simulink model "slexIonosphereClassificationSVMPredictExample"  (R2021a)
settings: Solver=FixedStepDiscrete  StartTime=0.0  StopTime=radarReturnInput.time(end)  RelTol=1e-3
PreLoadFcn:
  | load ionosphere
  | 
  | prsntX = X(1:300,:);
  | prsntY = Y(1:300);
  | ftrX = X(301:end,:);
  | ftrY = Y(301:end);
  | 
  | svmMdl = fitcsvm(prsntX,prsntY,'Standardize',true);
  | 
  | radarReturnInput.time = (0:50)';
  | radarReturnInput.signals(1).values = ftrX;
  | radarReturnInput.signals(1).dimensions = size(ftrX,2);
values from neighbouring files (symbols this model uses):
  X = meas(:,1:2)    [ClusteringUsingGaussianMixtureModelsExample.m]    (also in ComputePairwiseDistance2UsingACustomDistanceFunctionExample.m = rand(3,3); EstimatePosteriorClassProbabilitiesECOCExample.m = X'; FittingGaussianProcessRegressionModelsToLargeDatasetsExample.m = [X,X.^2]; ModelswithCorrelatedandUncorrelatedRandomEffectsExample.m = [ones(406,1) Acceleration Horsepower])
  Y = tsne(X,'Algorithm','barneshut','NumPCAComponents',50)    [ChangeTsneSettingsExample.m]    (also in ComputePairwiseDistance2UsingACustomDistanceFunctionExample.m = [X(:,1:2) rand(3,1)]; TSNEOutputFunctionExample.m = tsne(meas,'Options',opts,'Algorithm','exact'); TuneGaussianMixtureModelsExample.m = zeros(n,1); VisualizeHighDimensionalDataUsingTSNEExample.m)
libraries: statsLibrary x1
settings Model: Creator=The MathWorks, Inc.  LastModifiedBy=The MathWorks, Inc.
settings SolverCC: AlgebraicLoopSolver=TrustRegion
settings DataIOCC: ExternalInput=radarReturnInput  LoadExternalInput=on
settings DebuggingCC: SFMachineParentedDataDiag=warning

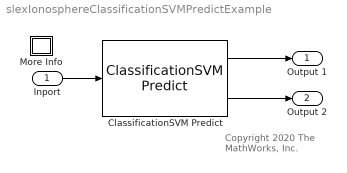
== system slexIonosphereClassificationSVMPredictExample ==
  note: Copyright 2020 The MathWorks, Inc.
  Inport : Inport  PortDimensions=34
  ClassificationSVM Predict : statsLibrary/Classification/ClassificationSVM Predict  TrainedLearner=svmMdl  ShowOutputScore=on  LabelOutMin=[]  LabelOutMax=[]  ScoreDataTypeStr=double  ScoreOutMin=[]  ScoreOutMax=[]  RawScoreDataTypeStr=double  RawScoreOutMin=[]  RawScoreOutMax=[]  KernelDataTypeStr=double  KernelOutMin=[]  KernelOutMax=[]  StoredEnumName=svmMdl_enumLabels
      settings: SourceProductBaseCode=ST
  More Info : Subsystem
      settings: OpenFcn=showExample('stats/PredictClassLabelsUsingClassificationSVMPredictBlockExample')
      mask Display: disp('?')
  Output 1 : Outport
  Output 2 : Outport  Port=2
  wires:
  Inport/1 -> ClassificationSVM Predict/1
  ClassificationSVM Predict/1 -> Output 1/1
  ClassificationSVM Predict/2 -> Output 2/1

== system slexIonosphereClassificationSVMPredictExample/More Info ==
